simulink model "SAD_project"  (R2023b)
settings: Solver=ode4  StartTime=t0  StopTime=tf  FixedStep=t_step  RelTol=1e-3
model workspace (MAT data in the model file):
  N_order = 1
values from neighbouring files (symbols this model uses):
  A1 = importdata("igrfSg.txt")    [SAD_project_code.m]
  A2 = importdata("igrfSh.txt")    [SAD_project_code.m]
  A_1 = area_face(1)    [SAD_project_code.m]
  A_2 = area_face(2)    [SAD_project_code.m]
  A_3 = area_face(3)    [SAD_project_code.m]
  A_4 = area_face(4)    [SAD_project_code.m]
  A_5 = area_face(5)    [SAD_project_code.m]
  A_6 = area_face(6)    [SAD_project_code.m]
  alpha = [1/6 5/6]    [SAD_project_code.m]
  ARW = ARW*[1 1 1]'    [SAD_project_code.m]
  bias = bias*[1 1 1]'    [SAD_project_code.m]
  DCM_eci_per = rotationMatrix(rad2deg(i),rad2deg(OM), rad2deg(om))    [SAD_project_code.m]
  e = 0.0011241    [SAD_project_code.m]
  FS = 50000e-9    (= 5e-05)    [SAD_project_code.m]
  H0 = [g_10 g_11 h_11]'    [SAD_project_code.m]
  h_r_0 = [0,0,0]'    [SAD_project_code.m]
  horizon_cone_limit = deg2rad(350)    [SAD_project_code.m]
  i = deg2rad(97.55)    [SAD_project_code.m]
  I = 5/12.*diag([Ix Iy Iz])    [SAD_project_code.m]
  I_inv = inv(I)    [SAD_project_code.m]
  I_RW = 1e-2    (= 0.01)    [SAD_project_code.m]
  I_vector_RW = [I_RW I_RW I_RW]'    [SAD_project_code.m]
  inc_tot = sqrt(inc_lin^2 + inc_acc^2)    [SAD_project_code.m]
  InitialTrueAnomalyOfEarth = 0    [SAD_project_code.m]
  j_b = [0.001 0.005 0.001]'    [SAD_project_code.m]
  matrix_RW_config = eye(3)    [SAD_project_code.m]
  matrix_RW_config_inv = inv(matrix_RW_config)    [SAD_project_code.m]
  mu_E = astroConstants(13)    [SAD_project_code.m]
  N_1 = BODY(1,:)    [SAD_project_code.m]
  N_2 = BODY(2,:)    [SAD_project_code.m]
  N_3 = BODY(3,:)    [SAD_project_code.m]
  N_4 = BODY(4,:)    [SAD_project_code.m]
  N_5 = BODY(5,:)    [SAD_project_code.m]
  N_6 = BODY(6,:)    [SAD_project_code.m]
  n_e = sqrt(mu_E/a^3)    [SAD_project_code.m]
  om = deg2rad(206.3209)    [SAD_project_code.m]
  OM = deg2rad(50.7464)    [SAD_project_code.m]
  p = a*(1-e^2)    [SAD_project_code.m]
  q0 = [0.1, -0.7, 0.51, 0.41]    [SAD_project_code.m]
  r_1 = r(1,:)    [SAD_project_code.m]
  r_2 = r(2,:)    [SAD_project_code.m]
  r_3 = r(3,:)    [SAD_project_code.m]
  r_4 = r(4,:)    [SAD_project_code.m]
  r_5 = r(5,:)    [SAD_project_code.m]
  r_6 = r(6,:)    [SAD_project_code.m]
  R_E = astroConstants(23)    [SAD_project_code.m]
  rho_d1 = 0.1    [SAD_project_code.m]
  rho_d2 = 0.1    [SAD_project_code.m]
  rho_d3 = 0.1    [SAD_project_code.m]
  rho_d4 = 0.1    [SAD_project_code.m]
  rho_d5 = 0.1    [SAD_project_code.m]
  rho_d6 = 0.1    [SAD_project_code.m]
  rho_s1 = rho_s(1)    [SAD_project_code.m]
  rho_s2 = rho_s(2)    [SAD_project_code.m]
  rho_s3 = rho_s(3)    [SAD_project_code.m]
  rho_s4 = rho_s(4)    [SAD_project_code.m]
  rho_s5 = rho_s(5)    [SAD_project_code.m]
  rho_s6 = rho_s(6)    [SAD_project_code.m]
  t_step = 0.01    [SAD_project_code.m]
  th0 = deg2rad(0)    [SAD_project_code.m]
  timeoflaunch = date2mjd2000(date0)    [SAD_project_code.m]
  ts_sensor = 5*t_step    (= 0.05)    [SAD_project_code.m]
  w0 = [wx0 wy0 wz0]'    [SAD_project_code.m]
  w0_RW = [0 0 0]    [SAD_project_code.m]
  w_E = deg2rad(15.04)/60/60    [SAD_project_code.m]
  wMax_RW = 2*pi * RPM_max_RW / 60    (= 527.263967027)    [SAD_project_code.m]
libraries: matrix_library x21, simulink x5, simulink_extras x4, dspindex x3, vrlib x2, aerolibutil x1
(part 1 of 3)
settings Model: Creator=samue  LastModifiedBy=rkomiii_masca

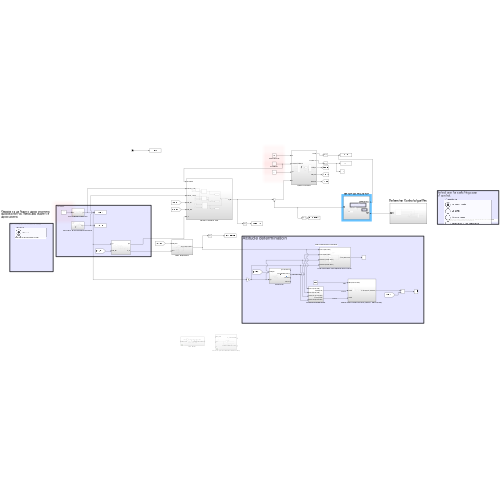
[thumbnail: Simulink's stored preview of the top-level diagram]
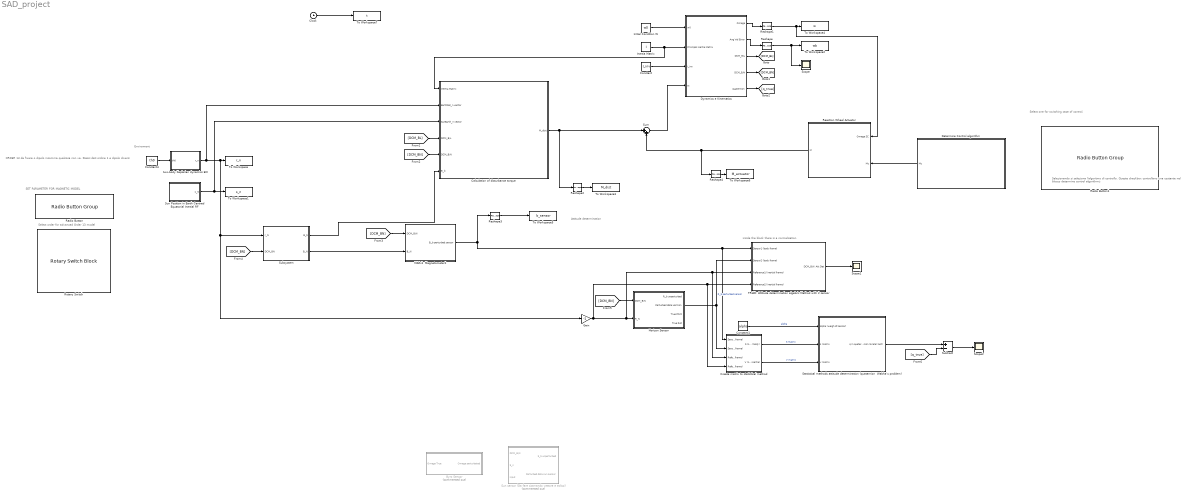
== system SAD_project ==
  note: ORDER 13 da fixare o dipolo insomma qualcosa non va. Stessi dati ordine 1 e dipolo diversi
  note: Select order for advanced Order 13 model
  note: SET PARAMETER FOR MAGNETIC MODEL
  note: Selezionando si seleziona l'algoritmo di controllo. Queste checkbox controllano una costante nel blocco determine control algorithmù
  note: Select one for switching case
      | of control.
  note: Attitude determination
  note: inside the block there is a normalisation
  note: Enviroment
  Calculation of disturbance torque : Subsystem
  Clock : Clock
  Constant : Constant  Value=I_inv
  Constant1 : Constant  Value=alpha
  Constant4 : Constant  Value=th0
  Create matrix to statistical method : Subsystem
  Determine Control algorithm : Subsystem
  Dynamics e Kinematics : Subsystem
  Gain : Gain  Gain=-1
  Gyro Sensor : Subsystem  Commented=on
  Horizon Sensor : Subsystem
  Inertia Matrix : Constant  Value=I  VectorParams1D=off
  Initial Condition W : Constant  Value=w0
  MAG-3  Magnetometer1 : Subsystem
  Radio Button : RadioButtonGroup  LabelPosition=Hide  SelectedLabel=Dipole model  ButtonGroupName=Magnetic field
      settings: Values={{'Dipole model', 'Order 13 model'}, [0 1]}
  Radio Button1 : RadioButtonGroup  LabelPosition=Hide  SelectedLabel=No control mode  ButtonGroupName=Control Mode
      settings: Values={{'No control mode', 'De-tumble', 'Slew maneuver', 'Pointing with 3 axis stabilization'}, [0 1 2 3]}
  Reaction Wheel Actuator : Subsystem
  Reshape{,1..4} (5 alike) : Reshape
  Rotary Switch : RotarySwitchBlock  LabelPosition=Hide
      settings: Values={{'1', '2', '3', '4', '5', '6', '7', '8', '9', '10', '11', '12', '13'}, [1 2 3 4 5 6 7 8 9 10 11 12 13]}
  Scope : Scope
  Scope1 : Scope
  Scope2 : Scope
  "Statistical methods attitude determination (quaternion  Wabha’s problem) " : Subsystem
  Subsystem : Subsystem
  Subtract : Sum  Inputs=+-
  Sum : Sum  Inputs=|++
  Sun Position in Earth Centred Equatorial Inertial RF : Subsystem
  Sun sensor (Da fare sistmando vettore e eclissi) : Subsystem  Commented=on
  TRIAD: Attitude determination algebric Method with 2 sensor : Subsystem
  To Workspace : ToWorkspace  VariableName=r_n  SampleTime=-1
  To Workspace1 : ToWorkspace  VariableName=s_n  SampleTime=-1
  To Workspace2 : ToWorkspace  VariableName=wb  SampleTime=-1
  To Workspace3 : ToWorkspace  VariableName=M_dist  SampleTime=-1
  To Workspace4 : ToWorkspace  VariableName=w  SampleTime=-1
  To Workspace5 : ToWorkspace  VariableName=b_sensor  SampleTime=-1
  To Workspace6 : ToWorkspace  VariableName=M_actuator  SampleTime=-1
  To Workspace7 : ToWorkspace  VariableName=t  SampleTime=-1
  two-body Keplerian dynamics ECI : Subsystem
  wires:
  two-body Keplerian dynamics ECI/1(r_n) -> Calculation of disturbance torque/2(EarthSat_n vector), Gain/1, Subsystem/1(r_N), To Workspace/1
  Inertia Matrix/1 -> Calculation of disturbance torque/1(Inertia Matrix), Dynamics e Kinematics/2(Principal Inertia Matrix)
  Initial Condition W/1 -> Dynamics e Kinematics/1(w0)
  Reshape/1 -> Scope/1, To Workspace2/1
  Dynamics e Kinematics/2(Ang Vel Error) -> Reshape/1
  Dynamics e Kinematics/3(DCM_B/L) -> [DCM_BL]
  Dynamics e Kinematics/1(Omega) -> Reshape1/1
  Constant4/1 -> two-body Keplerian dynamics ECI/1(th0)
  Constant/1 -> Dynamics e Kinematics/3(I_inv)
  Clock/1 -> To Workspace7/1
  Calculation of disturbance torque/1(M_dist) -> Sum/1, Reshape2/1
  [DCM_BN] -> MAG-3  Magnetometer1/1(DCM_B/N)
  [DCM_BL] -> Calculation of disturbance torque/4(DCM_B/L)
  [DCM_BN] -> Calculation of disturbance torque/5(DCM_B/N)
  [DCM_BN] -> Subsystem/2(DCM_BN)
  Reshape1/1 -> Reaction Wheel Actuator/1(Omega SC), To Workspace4/1
  Reshape2/1 -> To Workspace3/1
  Sun Position in Earth Centred Equatorial Inertial RF/1(s_N) -> To Workspace1/1, Calculation of disturbance torque/3(SunEarth_n vector)
  Dynamics e Kinematics/4(DCM_B/N) -> [DCM_BN]
  "Statistical methods attitude determination (quaternion  Wabha’s problem) "/1(q in quaternion (scalar last)) -> Subtract/1
  Create matrix to statistical method/2(V matrix (inertia)) -> "Statistical methods attitude determination (quaternion  Wabha’s problem) "/3(v matrix)  "V matrix"
  Constant1/1 -> "Statistical methods attitude determination (quaternion  Wabha’s problem) "/1(alpha (weigh of sensor))  "alpha"
  Create matrix to statistical method/1(S matrix (body)) -> "Statistical methods attitude determination (quaternion  Wabha’s problem) "/2(s matrix)  "S matrix"
  Horizon Sensor/2(Perturbed data Horizon) -> Create matrix to statistical method/2(Sensor2 (body frame)), TRIAD: Attitude determination algebric Method with 2 sensor/2(Sensor2 (body frame))  "R_b perturbed sensor"
  Gain/1 -> Horizon Sensor/2(R_N), TRIAD: Attitude determination algebric Method with 2 sensor/3(Reference1 (Inertial frame)), Create matrix to statistical method/3(Reference1 (Inertial frame)), TRIAD: Attitude determination algebric Method with 2 sensor/4(Reference2 (Inertial frame)), Create matrix to statistical method/4(Reference2 (Inertial frame))
  Reshape3/1 -> To Workspace5/1
  MAG-3  Magnetometer1/1(B_b perturbed sensor) -> Create matrix to statistical method/1(Sensor1 (body frame)), TRIAD: Attitude determination algebric Method with 2 sensor/1(Sensor1 (body frame)), Reshape3/1
  Subsystem/1(B_b) -> Calculation of disturbance torque/6(B_b)
  Determine Control algorithm/1(Mc) -> Reaction Wheel Actuator/2(Mc)
  Sum/1 -> Dynamics e Kinematics/4(M)
  Subsystem/2(B_N) -> MAG-3  Magnetometer1/2(B_N)
  [DCM_BN] -> Horizon Sensor/1(DCM_B/N)
  TRIAD: Attitude determination algebric Method with 2 sensor/1(DCM_B/N  Att Det) -> Scope1/1
  Dynamics e Kinematics/5(quaternion) -> [q_true]
  [q_true] -> Subtract/2
  Subtract/1 -> Scope2/1
  Reaction Wheel Actuator/1(M) -> Reshape4/1, Sum/2
  Reshape4/1 -> To Workspace6/1

== system SAD_project/Calculation of disturbance torque ==
  Inertia Matrix : Inport
  EarthSat_n vector : Inport  Port=2
  SunEarth_n vector : Inport  Port=3
  DCM_B/L : Inport  Port=4
  DCM_B/N : Inport  Port=5
  B_b : Inport  Port=6
  Extract Diagonal : matrix_library/Extract Diagonal
      settings: LibrarySourceBlock=|
      | simulink/Matrix
      | Operations/Extract Diagonal
  M of gravity gradient1 : Subsystem
  Magnetic Torque : Subsystem
  Reshape : Reshape
  Reshape1 : Reshape
  Solar pressure on 6 faces : Subsystem
  Sum : Sum  Inputs=|+++
  Terminator : Terminator
  To Workspace1 : ToWorkspace  VariableName=M_b  SampleTime=-1
  To Workspace3 : ToWorkspace  VariableName=M_GG  SampleTime=-1
  To Workspace8 : ToWorkspace  VariableName=M_SRP  SampleTime=-1
  j_b : Constant  Value=j_b
  M_dist : Outport
  wires:
  DCM_B/L/1 -> M of gravity gradient1/2(A_B/L)
  j_b/1 -> Magnetic Torque/1(j_b)
  Magnetic Torque/1(M_b) -> Sum/3, Reshape1/1
  B_b/1 -> Magnetic Torque/2(B_b)
  Inertia Matrix/1 -> Extract Diagonal/1
  DCM_B/N/1 -> Solar pressure on 6 faces/1(DCM)
  Sum/1 -> M_dist/1
  Reshape/1 -> To Workspace8/1
  Reshape1/1 -> To Workspace1/1
  M of gravity gradient1/1(GravityGradient_M) -> To Workspace3/1, Sum/1
  Solar pressure on 6 faces/2(Ftot_SP) -> Terminator/1
  Solar pressure on 6 faces/1(Mtot_SP) -> Reshape/1
  Extract Diagonal/1 -> M of gravity gradient1/1(Inertia Vector)
  EarthSat_n vector/1 -> Solar pressure on 6 faces/3("r_N "), M of gravity gradient1/3(r_N)
  SunEarth_n vector/1 -> Solar pressure on 6 faces/2(S_N)

== system SAD_project/Create matrix to statistical method ==
  Sensor1 (body frame) : Inport
  Sensor2 (body frame) : Inport  Port=2
  Reference1 (Inertial frame) : Inport  Port=3
  Reference2 (Inertial frame) : Inport  Port=4
  Matrix Concatenate1 : Concatenate  Mode=Multidimensional array  ConcatenateDimension=2
  Matrix Concatenate2 : Concatenate  Mode=Multidimensional array  ConcatenateDimension=2
  Normalize Vector1 : Subsystem
  Normalize Vector2 : Subsystem
  Normalize Vector3 : Subsystem
  Normalize Vector4 : Subsystem
  S matrix (body) : Outport
  V matrix (inertia) : Outport  Port=2
  wires:
  Matrix Concatenate1/1 -> V matrix (inertia)/1
  Normalize Vector1/1(Versor) -> Matrix Concatenate2/1
  Normalize Vector2/1(Versor) -> Matrix Concatenate2/2
  Normalize Vector4/1(Versor) -> Matrix Concatenate1/2
  Normalize Vector3/1(Versor) -> Matrix Concatenate1/1
  Matrix Concatenate2/1 -> S matrix (body)/1
  Reference1 (Inertial frame)/1 -> Normalize Vector3/1(Vector)
  Reference2 (Inertial frame)/1 -> Normalize Vector4/1(Vector)
  Sensor1 (body frame)/1 -> Normalize Vector1/1(Vector)
  Sensor2 (body frame)/1 -> Normalize Vector2/1(Vector)

== system SAD_project/Determine Control algorithm ==
  note: Modificare i case Switch case action tranquillamente aggiungendo tutti gli input desiderati
  Constant : Constant  Value=[1;1;1]
  Constant1 : Constant  Value=[2;2;2]
  Constant2 : Constant  Value=0
  Constant3 : Constant  Value=[3;3;3]
  Merge : Merge  Inputs=4
  Switch Case : SwitchCase  CaseConditions={1,2,3}
  Switch Case Action 3 axis stabilization Algorithm : Subsystem  TreatAsAtomicUnit=on
  Switch Case Action Detumle Algorithm : Subsystem  TreatAsAtomicUnit=on
  Switch Case Action Mc = 0 : Subsystem  TreatAsAtomicUnit=on
  Switch Case Action Slew Maneuver Algorithm : Subsystem  TreatAsAtomicUnit=on
  Mc : Outport
  wires:
  Switch Case/2 -> Switch Case Action Slew Maneuver Algorithm/Action  "slew maneuver"
  Switch Case/1 -> Switch Case Action Detumle Algorithm/Action  "Detumble case"
  Switch Case Action Slew Maneuver Algorithm/1(Out1) -> Merge/2
  Switch Case/3 -> Switch Case Action 3 axis stabilization Algorithm/Action  "pointing with 3 axis stabilization"
  Switch Case Action Mc = 0/1(Output) -> Merge/4
  Constant2/1 -> Switch Case/1
  Switch Case Action Detumle Algorithm/1(Output) -> Merge/1
  Switch Case Action 3 axis stabilization Algorithm/1(Out1) -> Merge/3
  Switch Case/4 -> Switch Case Action Mc = 0/Action  "Default: Contol moment == 0"
  Merge/1 -> Mc/1  "Control Moment"
  Constant/1 -> Switch Case Action Detumle Algorithm/1(Input)
  Constant1/1 -> Switch Case Action Slew Maneuver Algorithm/1(In1)
  Constant3/1 -> Switch Case Action 3 axis stabilization Algorithm/1(In1)

== system SAD_project/Dynamics e Kinematics ==
  w0 : Inport
  Principal Inertia Matrix : Inport  Port=2
  I_inv : Inport  Port=3
  M : Inport  Port=4
  Attitude error GG : Subsystem
  Constant6 : Constant  Value=q0
  DCM composition from quaternions 1 : Subsystem  AncestorBlock=LibrarySAD5/DCM composition from quaternions
  Kinematics quaternion2 : Subsystem
  Single spin dynamics : Subsystem  AncestorBlock=My_library/Single spin dynamics
  Terminator1 : Terminator
  Omega : Outport
  Ang Vel Error : Outport  Port=2
  DCM_B/L : Outport  Port=3
  DCM_B/N : Outport  Port=4
  quaternion : Outport  Port=5
  wires:
  DCM composition from quaternions 1/1(DCM) -> DCM_B/N/1, Attitude error GG/2(DCM_B/N)
  Constant6/1 -> Kinematics quaternion2/2(q0)
  Single spin dynamics/1(Omega) -> Omega/1, Attitude error GG/1(w), Kinematics quaternion2/1(omega)
  Kinematics quaternion2/2(q^(-1)) -> Terminator1/1
  M/1 -> Single spin dynamics/4(M)
  w0/1 -> Single spin dynamics/3(Omega_0)
  Principal Inertia Matrix/1 -> Single spin dynamics/2(Inertia matrix)
  Kinematics quaternion2/1(q) -> quaternion/1, DCM composition from quaternions 1/1(q(4x1))
  Attitude error GG/2(DCM_B/L) -> DCM_B/L/1
  Attitude error GG/1(Ang Vel Error) -> Ang Vel Error/1
  I_inv/1 -> Single spin dynamics/1(Inertia matrix inverse)

== system SAD_project/Gyro Sensor ==
  Omega True : Inport
  Band-Limited White Noise : simulink/Sources/Band-Limited White Noise  Cov=[0.00001]  Ts=0.1  seed=[23341]
  Constant : Constant  Value=ARW  VectorParams1D=off
  Constant1 : Constant  Value=bias  VectorParams1D=off
  Sum : Sum  Inputs=|++
  Sum1 : Sum  Inputs=|++
  Sum2 : Sum  Inputs=|++
  Zero-Order Hold : ZeroOrderHold  SampleTime=-1
  Omega perturbated : Outport
  wires:
  Zero-Order Hold/1 -> Sum/1
  Sum2/1 -> Omega perturbated/1
  Sum1/1 -> Sum2/1
  Sum/1 -> Sum1/1
  Omega True/1 -> Zero-Order Hold/1
  Constant1/1 -> Sum2/2
  Band-Limited White Noise/1 -> Sum/2
  Constant/1 -> Sum1/2

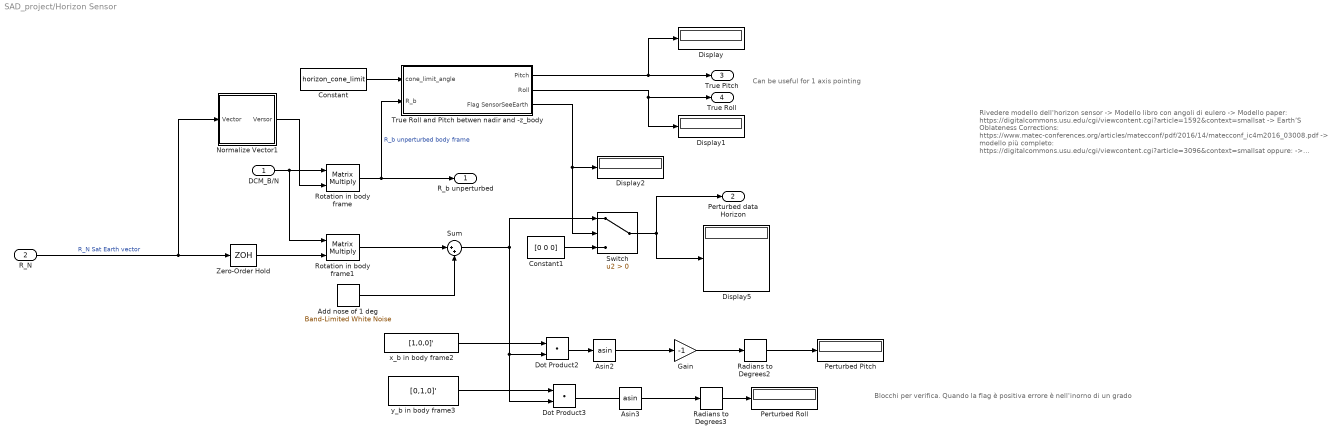
== system SAD_project/Horizon Sensor ==
  note: Can be useful for 1 axis pointing
  note: Rivedere modello dell'horizon sensor
      | -> Modello libro con angoli di eulero
      | -> Modello paper: https://digitalcommons.usu.edu/cgi/viewcontent.cgi?article=1592&context=smallsat
      | -> Earth’S Oblateness Corrections: https://www.matec-conferences.org/articles/matecconf/pdf/2016/14/matecconf_ic4m2016_03008.pdf
      | -> modello più completo: https://digitalcommons.usu.edu/cgi/viewcontent.cgi?article=3096&context=smallsat
      | oppure:
      | -> Sistemare errore in modo che non sia lineare
      | -> Controllare angoli e conversioni
  note: Blocchi per verifica. Quando la flag è positiva errore è nell'inorno di un grado
  DCM_B/N : Inport
  R_N : Inport  Port=2
  Add nose of 1 deg : simulink/Sources/Band-Limited White Noise  Cov=[0.000001 0.000001 0]  Ts=ts_sensor  seed=[23341]
  Asin2 : Trigonometry  Operator=asin
  Asin3 : Trigonometry  Operator=asin
  Constant : Constant  Value=horizon_cone_limit
  Constant1 : Constant  Value=[0 0 0]
  Display{,1..2,5} (4 alike) : Display
  Dot Product2 : DotProduct  OutDataTypeStr=Inherit: Inherit via internal rule
  Dot Product3 : DotProduct  OutDataTypeStr=Inherit: Inherit via internal rule
  Gain : Gain  Gain=-1
  Normalize Vector1 : Subsystem
  Perturbed Pitch : Display
  Perturbed Roll : Display
  Radians to Degrees2 : simulink_extras/Transformations/Radians to Degrees
  Radians to Degrees3 : simulink_extras/Transformations/Radians to Degrees
  Rotation in body frame : Product  Multiplication=Matrix(*)
  Rotation in body frame1 : Product  Multiplication=Matrix(*)
  Sum : Sum  Inputs=|++
  Switch : Switch  Criteria=u2 > Threshold  SaturateOnIntegerOverflow=off  InputSameDT=off
  True Roll and Pitch betwen nadir and -z_body : Subsystem
  Zero-Order Hold : ZeroOrderHold  SampleTime=ts_sensor
  x_b in body frame2 : Constant  Value=[1,0,0]'
  y_b in body frame3 : Constant  Value=[0,1,0]'
  R_b unperturbed : Outport
  Perturbed data Horizon : Outport  Port=2
  True Pitch : Outport  Port=3
  True Roll : Outport  Port=4
  wires:
  y_b in body frame3/1 -> Dot Product3/1
  Zero-Order Hold/1 -> Rotation in body frame1/2
  True Roll and Pitch betwen nadir and -z_body/3(Flag SensorSeeEarth) -> Switch/2, Display2/1
  Normalize Vector1/1(Versor) -> Rotation in body frame/2
  Rotation in body frame1/1 -> Sum/1
  Asin2/1 -> Gain/1
  DCM_B/N/1 -> Rotation in body frame/1, Rotation in body frame1/1
  Switch/1 -> Perturbed data Horizon/1, Display5/1
  True Roll and Pitch betwen nadir and -z_body/1(Pitch) -> Display/1, True Pitch/1
  Constant/1 -> True Roll and Pitch betwen nadir and -z_body/1(cone_limit_angle)
  Dot Product2/1 -> Asin2/1
  Rotation in body frame/1 -> R_b unperturbed/1, True Roll and Pitch betwen nadir and -z_body/2(R_b)  "R_b unperturbed body frame"
  Add nose of 1 deg/1 -> Sum/2
  True Roll and Pitch betwen nadir and -z_body/2(Roll) -> Display1/1, True Roll/1
  x_b in body frame2/1 -> Dot Product2/1
  Radians to Degrees2/1 -> Perturbed Pitch/1
  Sum/1 -> Switch/1, Dot Product2/2, Dot Product3/2
  Dot Product3/1 -> Asin3/1
  Asin3/1 -> Radians to Degrees3/1
  Gain/1 -> Radians to Degrees2/1
  Radians to Degrees3/1 -> Perturbed Roll/1
  Constant1/1 -> Switch/3
  R_N/1 -> Zero-Order Hold/1, Normalize Vector1/1(Vector)  "R_N Sat Earth vector"

== system SAD_project/MAG-3  Magnetometer1 ==
  note: CODE TO ADD TO MAKE SENSOR WORK
      | % Time definition
      | t0 = 0;
      | tf = T; %Period of orbit
      | t_step = 0.01; %fixed step of simulation
      | ts_sensor = t_step; % Sample of sensor (can change but must to be a multiple of t_step)
      |
      | % MAG-3 sensor data and error
      | FS = 500e-9; %Full scale value
      | inc_lin = 0.15/100; % Accuracy error
      | inc_acc = 0.75/100; % Linear error
      | inc_tot = sqrt(inc_lin^2 + inc_acc^2); %Total error
  DCM_B/N : Inport
  B_N : Inport  Port=2
  Error gain of sensor MAG-3 : Gain  Gain=inc_tot*FS
  Rotation in body frame : Product  Multiplication=Matrix(*)
  Saturation to FS : Saturate  UpperLimit=FS  LowerLimit=-FS
  Sum : Sum  Inputs=|++
  Vector Concatenate : Concatenate  NumInputs=3
  White Noise : RandomNumber  DisableCoverage=on  Seed=1  SampleTime=ts_sensor
  White Noise1 : RandomNumber  DisableCoverage=on  Seed=2  SampleTime=ts_sensor
  White Noise2 : RandomNumber  DisableCoverage=on  Seed=3  SampleTime=ts_sensor
  Zero-Order Hold : ZeroOrderHold  SampleTime=ts_sensor
  B_b perturbed sensor : Outport
  wires:
  Vector Concatenate/1 -> Error gain of sensor MAG-3/1
  White Noise/1 -> Vector Concatenate/1
  Error gain of sensor MAG-3/1 -> Sum/2
  White Noise2/1 -> Vector Concatenate/3
  White Noise1/1 -> Vector Concatenate/2
  DCM_B/N/1 -> Rotation in body frame/1
  B_N/1 -> Zero-Order Hold/1
  Zero-Order Hold/1 -> Rotation in body frame/2
  Saturation to FS/1 -> B_b perturbed sensor/1
  Rotation in body frame/1 -> Sum/1
  Sum/1 -> Saturation to FS/1

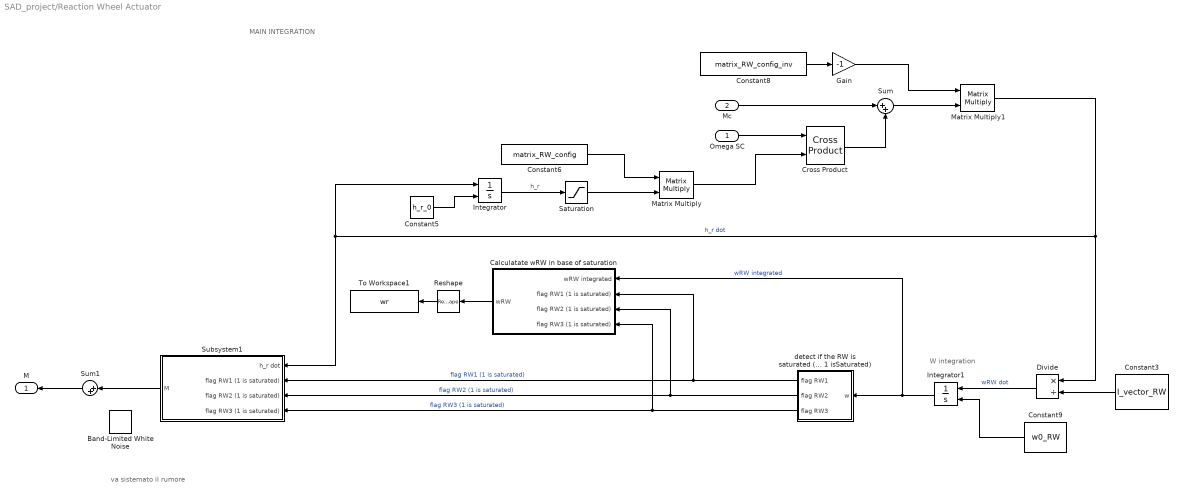
== system SAD_project/Reaction Wheel Actuator ==
  note: W integration
  note: va sistemato il rumore
  note: MAIN INTEGRATION
  Omega SC : Inport
  Mc : Inport  Port=2
  Band-Limited White Noise : simulink/Sources/Band-Limited White Noise  Cov=[0.00001, 0.00001, 0.00001]'  Ts=t_step  seed=[23341]
  Calculatate wRW in base of saturation : Subsystem
  Constant3 : Constant  Value=I_vector_RW
  Constant5 : Constant  Value=h_r_0  VectorParams1D=off
  Constant6 : Constant  Value=matrix_RW_config  VectorParams1D=off
  Constant8 : Constant  Value=matrix_RW_config_inv  VectorParams1D=off
  Constant9 : Constant  Value=w0_RW
  Cross Product : matrix_library/Cross Product
  Divide : Product  Inputs=*/
  Gain : Gain  Gain=-1
  Integrator : Integrator  InitialConditionSource=external
  Integrator1 : Integrator  InitialConditionSource=external
  Matrix Multiply : Product  Multiplication=Matrix(*)
  Matrix Multiply1 : Product  Multiplication=Matrix(*)
  Reshape : Reshape
  Saturation : Saturate  UpperLimit=wMax_RW*I_RW  LowerLimit=-wMax_RW*I_RW
  Subsystem1 : Subsystem
  Sum : Sum  Inputs=|++
  Sum1 : Sum  Inputs=|++
  To Workspace1 : ToWorkspace  VariableName=wr  SampleTime=-1
  detect if the RW is saturated (output == 1 isSaturated) : Subsystem
  M : Outport
  wires:
  Matrix Multiply1/1 -> Integrator/1, Subsystem1/1(h_r dot), Divide/1  "h_r dot"
  Constant6/1 -> Matrix Multiply/1
  Cross Product/1 -> Sum/2
  Constant8/1 -> Gain/1
  Sum/1 -> Matrix Multiply1/2
  detect if the RW is saturated (output == 1 isSaturated)/2(flag RW2) -> Calculatate wRW in base of saturation/3(flag RW2 (1 is saturated)), Subsystem1/3(flag RW2 (1 is saturated))  "flag RW2 (1 is saturated)"
  Calculatate wRW in base of saturation/1(wRW) -> Reshape/1
  Matrix Multiply/1 -> Cross Product/2
  Constant5/1 -> Integrator/2
  Constant3/1 -> Divide/2
  Gain/1 -> Matrix Multiply1/1
  Mc/1 -> Sum/1
  Saturation/1 -> Matrix Multiply/2
  Integrator1/1 -> Calculatate wRW in base of saturation/1(wRW integrated), detect if the RW is saturated (output == 1 isSaturated)/1(w)  "wRW integrated"
  Constant9/1 -> Integrator1/2
  Divide/1 -> Integrator1/1  "wRW dot"
  Integrator/1 -> Saturation/1  "h_r"
  detect if the RW is saturated (output == 1 isSaturated)/3(flag RW3) -> Calculatate wRW in base of saturation/4(flag RW3 (1 is saturated)), Subsystem1/4(flag RW3 (1 is saturated))  "flag RW3 (1 is saturated)"
  detect if the RW is saturated (output == 1 isSaturated)/1(flag RW1) -> Calculatate wRW in base of saturation/2(flag RW1 (1 is saturated)), Subsystem1/2(flag RW1 (1 is saturated))  "flag RW1 (1 is saturated)"
  Reshape/1 -> To Workspace1/1
  Omega SC/1 -> Cross Product/1
  Subsystem1/1(M) -> Sum1/1
  Sum1/1 -> M/1

== system SAD_project/Statistical methods attitude determination (quaternion  Wabha’s problem)  ==
  note: In questo blocco ci sono altri metodi per il calcolo di q
  note: BLOCCO DA SISTEMARE SCEGLIENDO UNA SOLUZIONE
  note: Resolve linear system:
      | (𝑆 − σI)𝑞 + zq_4 = 𝜆_(MAX)*𝑞
      | 𝑧'𝑞 + σ*q_4 = 𝜆_(MAX)*𝑞_4
      |
      | Calculate eigenvalue (in the theory we assumed that lambda_max = 1)
  note: 𝐾 = [ (𝑆 − σI), 𝑧
      | 𝑧 ' 𝜎 ]
  note: 𝑧 = [𝑏23 − 𝑏32 , b31 − 𝑏13 , b12 − 𝑏21] '
  alpha (weigh of sensor) : Inport
  s matrix : Inport  Port=2
  v matrix : Inport  Port=3
  Adjoint of 3x3 Matrix : aerolibutil/Adjoint of 3x3 Matrix
  Blocco da convertire in formato simulink. Ho trovato 3 soluzioni differenti al proble : MATLAB Function  TreatAsAtomicUnit=on
  For Iterator Subsystem to calculate B matrix : Subsystem  TreatAsAtomicUnit=on
  Gain : Gain  Gain=eye(3)
  Matrix Concatenate : Concatenate  Mode=Multidimensional array  ConcatenateDimension=2
  Matrix Concatenate1 : Concatenate  Mode=Multidimensional array
  Matrix trace : Subsystem
  Subtract : Sum  Inputs=+-
  Sum : Sum  Inputs=|++
  Transpose : Math  Operator=transpose
  Transpose2 : Math  Operator=transpose
  Vector Concatenate1 : Concatenate
  Vector z : Subsystem
  q in quaternion (scalar last) : Outport
  wires:
  Transpose/1 -> Sum/2
  For Iterator Subsystem to calculate B matrix/1(B matrix) -> Vector z/1(B), Matrix trace/1(Matrix), Transpose/1, Sum/1  "B matrix"
  Sum/1 -> Adjoint of 3x3 Matrix/1, Blocco da convertire in formato simulink. Ho trovato 3 soluzioni differenti al proble/2(S), Subtract/1  "matrix S"
  Gain/1 -> Subtract/2
  Matrix trace/1(trace) -> Vector Concatenate1/2, Gain/1  "sigma = tr(B)"
  Matrix Concatenate/1 -> Matrix Concatenate1/1
  Vector Concatenate1/1 -> Transpose2/1
  Vector z/1(z) -> Vector Concatenate1/1, Matrix Concatenate/2
  Transpose2/1 -> Matrix Concatenate1/2
  Subtract/1 -> Matrix Concatenate/1  "S - sigma*eye(3)"
  alpha (weigh of sensor)/1 -> For Iterator Subsystem to calculate B matrix/1(alpha)
  v matrix/1 -> For Iterator Subsystem to calculate B matrix/3(v matrix)
  s matrix/1 -> For Iterator Subsystem to calculate B matrix/2(s matrix)
  Blocco da convertire in formato simulink. Ho trovato 3 soluzioni differenti al proble/1(q) -> q in quaternion (scalar last)/1  "q in quaternion (scalar last)"
  Adjoint of 3x3 Matrix/1 -> Blocco da convertire in formato simulink. Ho trovato 3 soluzioni differenti al proble/3(Sadj)
  Matrix Concatenate1/1 -> Blocco da convertire in formato simulink. Ho trovato 3 soluzioni differenti al proble/1(K)  "K matrix"

== system SAD_project/Subsystem ==
  r_N : Inport
  DCM_BN : Inport  Port=2
  Control by check box : Constant  Value=0
  Matrix Multiply : Product  Multiplication=Matrix(*)
  Merge : Merge
  Reshape4 : Reshape
  Switch Case Action Adavanced Magnetic model : Subsystem  TreatAsAtomicUnit=on
  Switch Case Action Dipole model : Subsystem  TreatAsAtomicUnit=on
  Switch Case2 : SwitchCase
  To Workspace6 : ToWorkspace  VariableName=bn  SampleTime=-1
  B_b : Outport
  B_N : Outport  Port=2
  wires:
  Switch Case Action Dipole model/1(b_N) -> Merge/2
  Switch Case2/1 -> Switch Case Action Adavanced Magnetic model/Action
  Switch Case2/2 -> Switch Case Action Dipole model/Action
  Matrix Multiply/1 -> B_b/1
  DCM_BN/1 -> Matrix Multiply/1
  Control by check box/1 -> Switch Case2/1
  r_N/1 -> Switch Case Action Dipole model/1(r_N), Switch Case Action Adavanced Magnetic model/1(r_N)
  Switch Case Action Adavanced Magnetic model/1(B_n) -> Merge/1
  Reshape4/1 -> To Workspace6/1
  Merge/1 -> Reshape4/1, Matrix Multiply/2, B_N/1

== system SAD_project/Sun Position in Earth Centred Equatorial Inertial RF ==
  note: pointing Sun from Earth
      |
      | x=vernal line
      | y=perpendicular
      | z=cnp
  Clock : Clock
  Gain : Gain  Gain=cos(23.45/360*2*pi)
  Gain1 : Gain  Gain=sin(23.45/360*2*pi)
  InitialTrueAnomalyOfEarth : Constant  Value=InitialTrueAnomalyOfEarth
  MatrixMultiply : Product
  Mux : Mux  Inputs=3
  Product : Product
  Sum : Sum  Inputs=|++
  Trigonometric Function : Trigonometry  Operator=cos
  Trigonometric Function1 : Trigonometry
  mean ang vel : Constant  Value=2*pi/31536000
  mean distance : Constant  Value=149597870
  s_N : Outport
  wires:
  Trigonometric Function/1 -> Mux/1
  Gain1/1 -> Mux/3
  Mux/1 -> MatrixMultiply/2
  MatrixMultiply/1 -> s_N/1  "s_N"
  mean distance/1 -> MatrixMultiply/1
  Gain/1 -> Mux/2
  Trigonometric Function1/1 -> Gain1/1, Gain/1
  mean ang vel/1 -> Product/2
  Clock/1 -> Product/1
  InitialTrueAnomalyOfEarth/1 -> Sum/2
  Product/1 -> Sum/1
  Sum/1 -> Trigonometric Function1/1, Trigonometric Function/1

== system SAD_project/Sun sensor (Da fare sistmando vettore e eclissi) ==
  note: SUN SENSOR DA RIFINIRE, ma Utilizzabile
      | -> Modellare non rilevamento sole (esempio eclissi)
      | -> Modellare albedo terra/luna per riflessi
      | -> Sistemare distrubi basandosi su sensore reale
  DCM_B/N : Inport
  S_n : Inport  Port=2
  Input : Inport  Port=3
  Band-Limited White Noise : simulink/Sources/Band-Limited White Noise  Cov=5e9*[1 1 1]  Ts=ts_sensor  seed=[23341]
  Normalize Vector1 : Subsystem
  Rotation in body frame : Product  Multiplication=Matrix(*)
  Rotation in body frame1 : Product  Multiplication=Matrix(*)
  Sum : Sum  Inputs=|++
  Zero-Order Hold : ZeroOrderHold  SampleTime=ts_sensor
  S_b unperturbed : Outport
  Perturbed data sun sensor : Outport  Port=2
  wires:
  Band-Limited White Noise/1 -> Sum/2
  DCM_B/N/1 -> Rotation in body frame/1, Rotation in body frame1/1
  S_n/1 -> Zero-Order Hold/1, Normalize Vector1/1(Vector)
  Normalize Vector1/1(Versor) -> Rotation in body frame/2
  Zero-Order Hold/1 -> Rotation in body frame1/2
  Rotation in body frame1/1 -> Sum/1
  Rotation in body frame/1 -> S_b unperturbed/1
  Sum/1 -> Perturbed data sun sensor/1

== system SAD_project/TRIAD: Attitude determination algebric Method with 2 sensor ==
  note: 𝑉^(-1) = 𝑉';
      | 𝐴 = 𝑆𝑉^(-1) = 𝑆𝑉'
  note: 𝑣1 = 𝑎;
      | 𝑣2 = (𝑎 ∧ 𝑏)/|𝑎 ∧ 𝑏|;
      | 𝑣3 = 𝑎 ∧ 𝑣2
  note: S1 = 𝑝;
      | 𝑠2 = (𝑝 ∧ 𝑞)/(|𝑝 ∧ 𝑞|);
      | 𝑠3 = 𝑝 ∧ 𝑠2
  Sensor1 (body frame) : Inport
  Sensor2 (body frame) : Inport  Port=2
  Reference1 (Inertial frame) : Inport  Port=3
  Reference2 (Inertial frame) : Inport  Port=4
  Matrix Multiply : Product  Multiplication=Matrix(*)
  Normalize Vector1 : Subsystem
  Normalize Vector2 : Subsystem
  Normalize Vector3 : Subsystem
  Normalize Vector4 : Subsystem
  Subsystem : Subsystem
  Subsystem1 : Subsystem
  Transpose : Math  Operator=transpose
  DCM_B/N  Att Det : Outport
  wires:
  Sensor1 (body frame)/1 -> Normalize Vector2/1(Vector)  "q"
  Sensor2 (body frame)/1 -> Normalize Vector3/1(Vector)  "p"
  Subsystem/1("Matrix S Measurements ") -> Matrix Multiply/1  "Matrix S Measurements (body frame)"
  Normalize Vector2/1(Versor) -> Subsystem/1(versor p (body frame))
  Normalize Vector3/1(Versor) -> Subsystem/2(versor q (body frame))
  Normalize Vector1/1(Versor) -> Subsystem1/1(versor a (body frame))
  Reference2 (Inertial frame)/1 -> Normalize Vector4/1(Vector)  "b"
  Reference1 (Inertial frame)/1 -> Normalize Vector1/1(Vector)  "a"
  Subsystem1/1("Matrix V certain model ") -> Transpose/1  "Matrix V (inertial frame)"
  Normalize Vector4/1(Versor) -> Subsystem1/2(versor b (body frame))
  Matrix Multiply/1 -> DCM_B/N  Att Det/1  "DCM_B/N from attirude determination"
  Transpose/1 -> Matrix Multiply/2

== system SAD_project/two-body Keplerian dynamics ECI ==
  th0 : Inport
  Constant : Constant  Value=DCM_eci_per
  Integretion of true anomaly : Subsystem
  Matrix Multiply : Product  Multiplication=Matrix(*)
  Transpose : Math  Operator=transpose
  r_perifocal : Subsystem
  r_n : Outport
  wires:
  th0/1 -> Integretion of true anomaly/1(th0)
  Integretion of true anomaly/1(th) -> r_perifocal/1(th)
  Constant/1 -> Transpose/1
  Transpose/1 -> Matrix Multiply/1
  r_perifocal/1(r_per) -> Matrix Multiply/2
  Matrix Multiply/1 -> r_n/1

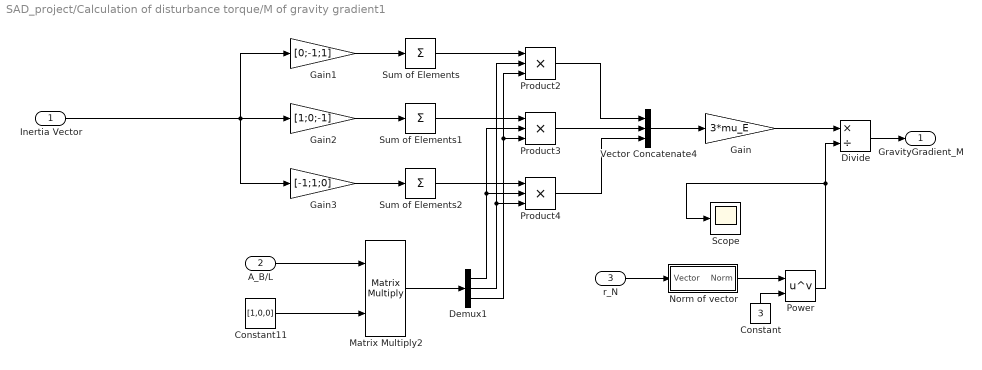
== system SAD_project/Calculation of disturbance torque/M of gravity gradient1 ==
  Inertia Vector : Inport
  A_B/L : Inport  Port=2
  r_N : Inport  Port=3
  Constant : Constant  Value=3
  Constant11 : Constant  Value=[1,0,0]
  Demux1 : Demux  Outputs=3
  Divide : Product  Inputs=*/
  Gain : Gain  Gain=3*mu_E
  Gain1 : Gain  Gain=[0;-1;1]
  Gain2 : Gain  Gain=[1;0;-1]
  Gain3 : Gain  Gain=[-1;1;0]
  Matrix Multiply2 : Product  Multiplication=Matrix(*)
  Norm of vector : Subsystem  AncestorBlock=LibrarySAD5/Normalize Vector1
  Power : Math  Operator=pow
  Product2 : Product  Inputs=3
  Product3 : Product  Inputs=3
  Product4 : Product  Inputs=3
  Scope : Scope
  Sum of Elements : Sum  Inputs=+
  Sum of Elements1 : Sum  Inputs=+
  Sum of Elements2 : Sum  Inputs=+
  Vector Concatenate4 : Concatenate  NumInputs=3
  GravityGradient_M : Outport
  wires:
  Demux1/3 -> Product2/3, Product3/3
  Product2/1 -> Vector Concatenate4/1
  Matrix Multiply2/1 -> Demux1/1
  Product4/1 -> Vector Concatenate4/3
  Product3/1 -> Vector Concatenate4/2
  Demux1/1 -> Product4/2, Product3/2
  Constant11/1 -> Matrix Multiply2/2
  Demux1/2 -> Product4/3, Product2/2
  A_B/L/1 -> Matrix Multiply2/1
  Vector Concatenate4/1 -> Gain/1
  Gain1/1 -> Sum of Elements/1
  Gain2/1 -> Sum of Elements1/1
  Gain3/1 -> Sum of Elements2/1
  Sum of Elements/1 -> Product2/1
  Sum of Elements1/1 -> Product3/1
  Sum of Elements2/1 -> Product4/1
  Inertia Vector/1 -> Gain1/1, Gain2/1, Gain3/1
  Gain/1 -> Divide/1
  Power/1 -> Scope/1, Divide/2
  Constant/1 -> Power/2
  r_N/1 -> Norm of vector/1(Vector)
  Divide/1 -> GravityGradient_M/1
  Norm of vector/1(Norm) -> Power/1

== system SAD_project/Calculation of disturbance torque/Magnetic Torque ==
  j_b : Inport
  B_b : Inport  Port=2
  Cross Product : matrix_library/Cross Product
  M_b : Outport
  wires:
  Cross Product/1 -> M_b/1
  j_b/1 -> Cross Product/1
  B_b/1 -> Cross Product/2

== system SAD_project/Calculation of disturbance torque/Solar pressure on 6 faces ==
  DCM : Inport
  S_N : Inport  Port=2
  "r_N " : Inport  Port=3
  Acos : Trigonometry  Operator=acos
  Dot Product : DotProduct  OutDataTypeStr=Inherit: Inherit via internal rule
  MatrixMultiply : Product  Multiplication=Matrix(*)
  MatrixMultiply1 : Product  Multiplication=Matrix(*)
  Norm of vector : Subsystem  AncestorBlock=LibrarySAD5/Normalize Vector1
  Normalize Vector : vrlib/Utilities/Normalize Vector  maxzero=0
  Normalize Vector1 : vrlib/Utilities/Normalize Vector  maxzero=0
  Solar pressure on 6 faces1 : Subsystem
  Sum1 : Sum  Inputs=|+-
  Mtot_SP : Outport
  Ftot_SP : Outport  Port=2
  wires:
  DCM/1 -> MatrixMultiply1/1, MatrixMultiply/1
  S_N/1 -> Norm of vector/1(Vector), Sum1/1, MatrixMultiply/2, Normalize Vector1/1
  "r_N "/1 -> Sum1/2, MatrixMultiply1/2
  MatrixMultiply1/1 -> Solar pressure on 6 faces1/2(r_B)
  Norm of vector/1(Norm) -> Solar pressure on 6 faces1/5(s_N norm)
  MatrixMultiply/1 -> Solar pressure on 6 faces1/1(s_B)
  Sum1/1 -> Solar pressure on 6 faces1/4(S_N - r_N), Normalize Vector/1
  Normalize Vector/1 -> Dot Product/1
  Normalize Vector1/1 -> Dot Product/2
  Solar pressure on 6 faces1/1(Ftot_SP) -> Ftot_SP/1
  Dot Product/1 -> Acos/1
  Acos/1 -> Solar pressure on 6 faces1/3(S/E_S/sc_angle)
  Solar pressure on 6 faces1/2(Mtot_SP) -> Mtot_SP/1

== system SAD_project/Create matrix to statistical method/Normalize Vector1 ==
  Vector : Inport
  Divide : Product  Inputs=*/
  Normalize Vector : Subsystem  AncestorBlock=LibrarySAD5/Normalize Vector1
  Versor : Outport
  wires:
  Vector/1 -> Normalize Vector/1(Vector), Divide/1
  Divide/1 -> Versor/1
  Normalize Vector/1(Norm) -> Divide/2

== system SAD_project/Create matrix to statistical method/Normalize Vector2 ==
  Vector : Inport
  Divide : Product  Inputs=*/
  Normalize Vector : Subsystem  AncestorBlock=LibrarySAD5/Normalize Vector1
  Versor : Outport
  wires:
  Vector/1 -> Normalize Vector/1(Vector), Divide/1
  Divide/1 -> Versor/1
  Normalize Vector/1(Norm) -> Divide/2

== system SAD_project/Create matrix to statistical method/Normalize Vector3 ==
  Vector : Inport
  Divide : Product  Inputs=*/
  Normalize Vector : Subsystem  AncestorBlock=LibrarySAD5/Normalize Vector1
  Versor : Outport
  wires:
  Vector/1 -> Normalize Vector/1(Vector), Divide/1
  Divide/1 -> Versor/1
  Normalize Vector/1(Norm) -> Divide/2

== system SAD_project/Create matrix to statistical method/Normalize Vector4 ==
  Vector : Inport
  Divide : Product  Inputs=*/
  Normalize Vector : Subsystem  AncestorBlock=LibrarySAD5/Normalize Vector1
  Versor : Outport
  wires:
  Vector/1 -> Normalize Vector/1(Vector), Divide/1
  Divide/1 -> Versor/1
  Normalize Vector/1(Norm) -> Divide/2

== system SAD_project/Determine Control algorithm/Switch Case Action 3 axis stabilization Algorithm ==
  In1 : Inport
  Action Port : ActionPort  ActionPortLabel=case [ 3 ]:
  Out1 : Outport
  wires:
  In1/1 -> Out1/1

== system SAD_project/Determine Control algorithm/Switch Case Action Detumle Algorithm ==
  Input : Inport
  Action Port : ActionPort  PropagateVarSize=During execution  ActionPortLabel=case [ 1 ]:
  Output : Outport
  wires:
  Input/1 -> Output/1

== system SAD_project/Determine Control algorithm/Switch Case Action Mc = 0 ==
  Action Port : ActionPort  PropagateVarSize=During execution  ActionPortLabel=default:
  Constant : Constant  Value=[0 0 0]'
  Output : Outport
  wires:
  Constant/1 -> Output/1

== system SAD_project/Determine Control algorithm/Switch Case Action Slew Maneuver Algorithm ==
  In1 : Inport
  Action Port : ActionPort  ActionPortLabel=case [ 2 ]:
  Out1 : Outport
  wires:
  In1/1 -> Out1/1

== system SAD_project/Dynamics e Kinematics/Attitude error GG ==
  w : Inport
  DCM_B/N : Inport  Port=2
  Clock : Clock
  Constant : Constant  Value=n_e
  Constant5 : Constant  Value=0
  Matrix Multiply1 : Product  Multiplication=Matrix(*)
  Product : Product
  Subtract : Sum  Inputs=+-
  Vector Concatenate3 : Concatenate  NumInputs=3
  calculating A_B/L : Subsystem
  Ang Vel Error : Outport
  DCM_B/L : Outport  Port=2
  wires:
  Constant5/1 -> Vector Concatenate3/2, Vector Concatenate3/1
  Vector Concatenate3/1 -> Matrix Multiply1/2  "w_L/N"
  calculating A_B/L/1(A_B/L) -> Matrix Multiply1/1, DCM_B/L/1
  Matrix Multiply1/1 -> Subtract/2  "A_B/L * w_L/N"
  w/1 -> Subtract/1
  Subtract/1 -> Ang Vel Error/1
  Product/1 -> calculating A_B/L/1(Theta)  "Theta"
  Clock/1 -> Product/2
  Constant/1 -> Product/1, Vector Concatenate3/3
  DCM_B/N/1 -> calculating A_B/L/2(A_B/N)

== system SAD_project/Dynamics e Kinematics/DCM composition from quaternions 1 ==
  q(4x1) : Inport
  Cross product matrix composition : Subsystem
  Demux : Demux
  Dot Product : DotProduct  OutDataTypeStr=Inherit: Inherit via internal rule
  Gain : Gain  Gain=[1 0 0; 0 1 0; 0 0 1]
  Gain1 : Gain  Gain=2
  Gain2 : Gain  Gain=-2
  Mux : Mux  Inputs=3
  Product : Product  Multiplication=Matrix(*)
  Product1 : Product
  Square : Math  Operator=square
  Sum : Sum  Inputs=|-+
  Sum1 : Sum  Inputs=+++
  Transpose : Math  Operator=transpose
  DCM : Outport
  wires:
  Gain/1 -> Sum1/1
  Demux/1 -> Mux/1
  q(4x1)/1 -> Demux/1
  Demux/2 -> Mux/2
  Mux/1 -> Dot Product/2, Dot Product/1, Product/1, Cross product matrix composition/1(q_vect), Transpose/1  "q_vect"
  Demux/4 -> Gain2/1, Square/1  "q4"
  Demux/3 -> Mux/3
  Dot Product/1 -> Sum/1
  Sum/1 -> Gain/1
  Square/1 -> Sum/2
  Transpose/1 -> Product/2
  Product/1 -> Gain1/1
  Gain2/1 -> Product1/2
  Cross product matrix composition/1(q_vect cross) -> Product1/1  "omega_mat"
  Product1/1 -> Sum1/3
  Gain1/1 -> Sum1/2
  Sum1/1 -> DCM/1

== system SAD_project/Dynamics e Kinematics/Kinematics quaternion2 ==
  omega : Inport
  q0 : Inport  Port=2
  Demux : Demux
  Divide : Product  Inputs=*/
  Gain1 : Gain  Gain=-1
  Gain2 : Gain  Gain=-1
  Gain3 : Gain  Gain=1/2
  Gain4 : Gain  Gain=-1
  Integrator : Integrator  InitialConditionSource=external
  Matrix Multiply : Product  Multiplication=Matrix(*)
  Matrix OMEGA : Subsystem
  Mux : Mux
  Normalize Vector2 : Subsystem
  q : Outport
  q^(-1) : Outport  Port=2
  wires:
  Gain3/1 -> Matrix Multiply/1
  Matrix Multiply/1 -> Integrator/1
  omega/1 -> Matrix OMEGA/1(omega)
  Integrator/1 -> Normalize Vector2/1(Vector), Divide/1, Demux/1, q/1
  Matrix OMEGA/1(Matrix Omega) -> Gain3/1
  q0/1 -> Integrator/2
  Demux/2 -> Gain1/1
  Demux/3 -> Gain2/1
  Demux/4 -> Gain4/1
  Gain1/1 -> Mux/2
  Gain2/1 -> Mux/3
  Gain4/1 -> Mux/4
  Demux/1 -> Mux/1
  Mux/1 -> q^(-1)/1
  Normalize Vector2/1(Norm) -> Divide/2
  Divide/1 -> Matrix Multiply/2

== system SAD_project/Dynamics e Kinematics/Single spin dynamics ==
  Inertia matrix inverse : Inport
  Inertia matrix : Inport  Port=2
  Omega_0 : Inport  Port=3
  M : Inport  Port=4
  Cross Product : matrix_library/Cross Product
  Integrator1 : Integrator  InitialConditionSource=external
  Product : Product  Multiplication=Matrix(*)
  Product1 : Product  Multiplication=Matrix(*)
  Scope2 : Scope
  Sum : Sum  Inputs=|++
  Transpose1 : Math  Operator=transpose
  Omega : Outport
  wires:
  Transpose1/1 -> Omega/1
  Inertia matrix inverse/1 -> Product/1
  Integrator1/1 -> Product1/2, Transpose1/1, Cross Product/2, Scope2/1  "omega"
  Product/1 -> Integrator1/1  "omega_dot"
  Omega_0/1 -> Integrator1/2
  Product1/1 -> Cross Product/1
  Inertia matrix/1 -> Product1/1
  Cross Product/1 -> Sum/1
  Sum/1 -> Product/2
  M/1 -> Sum/2

== system SAD_project/Horizon Sensor/Normalize Vector1 ==
  Vector : Inport
  Divide : Product  Inputs=*/
  Normalize Vector : Subsystem  AncestorBlock=LibrarySAD5/Normalize Vector1
  Versor : Outport
  wires:
  Vector/1 -> Normalize Vector/1(Vector), Divide/1
  Divide/1 -> Versor/1
  Normalize Vector/1(Norm) -> Divide/2

== system SAD_project/Horizon Sensor/True Roll and Pitch betwen nadir and -z_body ==
  cone_limit_angle : Inport
  R_b : Inport  Port=2
  Abs : Abs  SaturateOnIntegerOverflow=off
  Abs1 : Abs  SaturateOnIntegerOverflow=off
  Asin : Trigonometry  Operator=asin
  Asin1 : Trigonometry  Operator=asin
  By defintion : Gain  Gain=-1
  Dot Product : DotProduct  OutDataTypeStr=Inherit: Inherit via internal rule
  Dot Product1 : DotProduct  OutDataTypeStr=Inherit: Inherit via internal rule
  Equal : RelationalOperator  Operator=>  OutDataTypeStr=boolean  RndMeth=Simplest  InputSameDT=off
  Equal1 : RelationalOperator  Operator=>  OutDataTypeStr=boolean  RndMeth=Simplest  InputSameDT=off
  NOT : Logic  Operator=NOT  IconShape=distinctive  AllPortsSameDT=off  OutDataTypeStr=boolean
  OR : Logic  Operator=OR  IconShape=distinctive  AllPortsSameDT=off  OutDataTypeStr=boolean
  Radians to Degrees : simulink_extras/Transformations/Radians to Degrees
  Radians to Degrees1 : simulink_extras/Transformations/Radians to Degrees
  x_b in body frame : Constant  Value=[1,0,0]'
  y_b in body frame1 : Constant  Value=[0,1,0]'
  Pitch : Outport
  Roll : Outport  Port=2
  Flag SensorSeeEarth : Outport  Port=3
  wires:
  Equal/1 -> OR/1
  Dot Product1/1 -> Asin1/1
  R_b/1 -> Dot Product1/2, Dot Product/2
  x_b in body frame/1 -> Dot Product/1
  y_b in body frame1/1 -> Dot Product1/1
  Dot Product/1 -> Asin/1
  By defintion/1 -> Radians to Degrees/1, Abs/1
  Asin/1 -> By defintion/1
  Asin1/1 -> Abs1/1, Radians to Degrees1/1
  Radians to Degrees1/1 -> Roll/1
  Abs1/1 -> Equal1/1
  Radians to Degrees/1 -> Pitch/1
  Abs/1 -> Equal/1
  cone_limit_angle/1 -> Equal/2, Equal1/2  "cone max angle"
  Equal1/1 -> OR/2
  OR/1 -> NOT/1
  NOT/1 -> Flag SensorSeeEarth/1

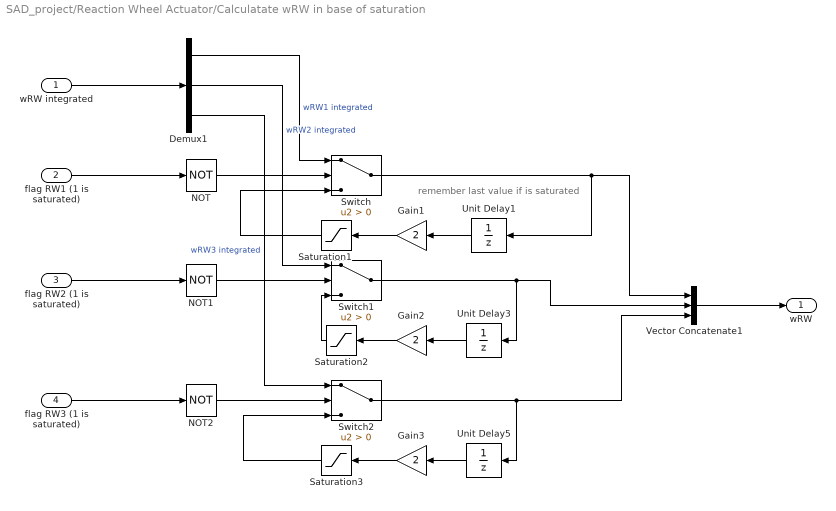
== system SAD_project/Reaction Wheel Actuator/Calculatate wRW in base of saturation ==
  note: remember last value if is saturated
  wRW integrated : Inport
  flag RW1 (1 is saturated) : Inport  Port=2
  flag RW2 (1 is saturated) : Inport  Port=3
  flag RW3 (1 is saturated) : Inport  Port=4
  Demux1 : Demux  Outputs=3
  Gain1 : Gain  Gain=2
  Gain2 : Gain  Gain=2
  Gain3 : Gain  Gain=2
  NOT : Logic  Operator=NOT  IconShape=distinctive  AllPortsSameDT=off  OutDataTypeStr=boolean
  NOT1 : Logic  Operator=NOT  IconShape=distinctive  AllPortsSameDT=off  OutDataTypeStr=boolean
  NOT2 : Logic  Operator=NOT  IconShape=distinctive  AllPortsSameDT=off  OutDataTypeStr=boolean
  Saturation1 : Saturate  UpperLimit=wMax_RW  LowerLimit=-wMax_RW
  Saturation2 : Saturate  UpperLimit=wMax_RW  LowerLimit=-wMax_RW
  Saturation3 : Saturate  UpperLimit=wMax_RW  LowerLimit=-wMax_RW
  Switch : Switch  Criteria=u2 > Threshold  SaturateOnIntegerOverflow=off  InputSameDT=off
  Switch1 : Switch  Criteria=u2 > Threshold  SaturateOnIntegerOverflow=off  InputSameDT=off
  Switch2 : Switch  Criteria=u2 > Threshold  SaturateOnIntegerOverflow=off  InputSameDT=off
  Unit Delay1 : UnitDelay  SampleTime=-1  HasFrameUpgradeWarning=on
  Unit Delay3 : UnitDelay  SampleTime=-1  HasFrameUpgradeWarning=on
  Unit Delay5 : UnitDelay  SampleTime=-1  HasFrameUpgradeWarning=on
  Vector Concatenate1 : Concatenate  NumInputs=3
  wRW : Outport
  wires:
  Gain2/1 -> Saturation2/1
  Switch1/1 -> Unit Delay3/1, Vector Concatenate1/2
  NOT/1 -> Switch/2
  flag RW1 (1 is saturated)/1 -> NOT/1
  Saturation3/1 -> Switch2/3
  NOT1/1 -> Switch1/2
  Saturation2/1 -> Switch1/3
  wRW integrated/1 -> Demux1/1
  Switch2/1 -> Unit Delay5/1, Vector Concatenate1/3
  Unit Delay5/1 -> Gain3/1
  Unit Delay3/1 -> Gain2/1
  Demux1/2 -> Switch1/1  "wRW2 integrated"
  Gain1/1 -> Saturation1/1
  Vector Concatenate1/1 -> wRW/1
  Switch/1 -> Unit Delay1/1, Vector Concatenate1/1
  Unit Delay1/1 -> Gain1/1
  Saturation1/1 -> Switch/3
  Demux1/3 -> Switch2/1  "wRW3 integrated"
  Demux1/1 -> Switch/1  "wRW1 integrated"
  NOT2/1 -> Switch2/2
  Gain3/1 -> Saturation3/1
  flag RW3 (1 is saturated)/1 -> NOT2/1
  flag RW2 (1 is saturated)/1 -> NOT1/1

== system SAD_project/Reaction Wheel Actuator/Subsystem1 ==
  h_r dot : Inport
  flag RW1 (1 is saturated) : Inport  Port=2
  flag RW2 (1 is saturated) : Inport  Port=3
  flag RW3 (1 is saturated) : Inport  Port=4
  Constant10 : Constant  Value=0
  Constant11 : Constant  Value=0
  Constant7 : Constant  Value=0
  Demux3 : Demux  Outputs=3
  Switch1 : Switch  Criteria=u2 > Threshold  SaturateOnIntegerOverflow=off  InputSameDT=off
  Switch2 : Switch  Criteria=u2 > Threshold  SaturateOnIntegerOverflow=off  InputSameDT=off
  Switch3 : Switch  Criteria=u2 > Threshold  SaturateOnIntegerOverflow=off  InputSameDT=off
  Vector Concatenate2 : Concatenate  NumInputs=3
  M : Outport
  wires:
  Demux3/3 -> Switch2/3
  Constant11/1 -> Switch2/1
  Switch2/1 -> Vector Concatenate2/3
  Demux3/1 -> Switch3/3
  Demux3/2 -> Switch1/3
  Switch3/1 -> Vector Concatenate2/1
  Switch1/1 -> Vector Concatenate2/2
  flag RW3 (1 is saturated)/1 -> Switch2/2
  Constant7/1 -> Switch3/1
  Constant10/1 -> Switch1/1
  flag RW1 (1 is saturated)/1 -> Switch3/2
  h_r dot/1 -> Demux3/1
  flag RW2 (1 is saturated)/1 -> Switch1/2
  Vector Concatenate2/1 -> M/1

== system SAD_project/Reaction Wheel Actuator/detect if the RW is saturated (output == 1 isSaturated) ==
  w : Inport
  Abs : Abs  SaturateOnIntegerOverflow=off
  Compare To Constant : simulink/Logic and Bit Operations/Compare To Constant  relop=>=  const=wMax_RW  OutDataTypeStr=boolean
  Demux : Demux  Outputs=3
  Logical Operator : Logic  Operator=OR  AllPortsSameDT=off  OutDataTypeStr=boolean
  Logical Operator1 : Logic  Operator=OR  AllPortsSameDT=off  OutDataTypeStr=boolean
  Logical Operator2 : Logic  Operator=OR  AllPortsSameDT=off  OutDataTypeStr=boolean
  Unit Delay : UnitDelay  SampleTime=-1  HasFrameUpgradeWarning=on
  Unit Delay2 : UnitDelay  SampleTime=-1  HasFrameUpgradeWarning=on
  Unit Delay4 : UnitDelay  SampleTime=-1  HasFrameUpgradeWarning=on
  flag RW1 : Outport
  flag RW2 : Outport  Port=2
  flag RW3 : Outport  Port=3
  wires:
  Unit Delay4/1 -> Logical Operator2/2
  Unit Delay/1 -> Logical Operator/2
  Demux/1 -> Logical Operator/1
  Logical Operator/1 -> flag RW1/1, Unit Delay/1
  Unit Delay2/1 -> Logical Operator1/2
  Logical Operator2/1 -> flag RW3/1, Unit Delay4/1
  Demux/2 -> Logical Operator1/1
  Logical Operator1/1 -> flag RW2/1, Unit Delay2/1
  Demux/3 -> Logical Operator2/1
  Abs/1 -> Compare To Constant/1
  w/1 -> Abs/1
  Compare To Constant/1 -> Demux/1

== system SAD_project/Statistical methods attitude determination (quaternion  Wabha’s problem) /For Iterator Subsystem to calculate B matrix ==
  note: Remember the last matrix B
  note: count the index
      | Important to flag reset in "State variable" to reset unit delay
  note: It's a for loop that resolve this expression
      | 𝐵 = ∑ 𝛼_𝑖*𝑠_𝑖*𝑣_𝑖' = [𝑏ij] to obatain matix B that it is a square matrix of order 3
      |
      | Analogous code for the iteration:
      |
      | for i = 1:size(alpha,2)
      | B = B + alpha(i)*s(:,i)*v(:,i)'
      | end
  alpha : Inport
  s matrix : Inport  Port=2
  v matrix : Inport  Port=3
  Add : Sum
  For Iterator : ForIterator  ResetStates=reset  IterationLimit=size(alpha,2)
  Matrix Multiply : Product  Multiplication=Matrix(*)
  Product : Product
  Transpose : Math  Operator=transpose
  Unit Delay1 : UnitDelay  SampleTime=-1  HasFrameUpgradeWarning=on
  Variable Selector : dspindex/Variable Selector  NumInputs=1  rowsOrCols=Columns  IdxMode=Variable  Elements=[1 3]  ZerOneIdxMode=One-based  errmode=Clip Index  FillMode=on  FillValues=0
  Variable Selector1 : dspindex/Variable Selector  NumInputs=1  rowsOrCols=Columns  IdxMode=Variable  Elements=[1 3]  ZerOneIdxMode=One-based  errmode=Clip Index  FillMode=on  FillValues=0
  Variable Selector2 : dspindex/Variable Selector  NumInputs=1  rowsOrCols=Columns  IdxMode=Variable  Elements=[1 3]  ZerOneIdxMode=One-based  errmode=Clip Index  FillMode=on  FillValues=0
  B matrix : Outport
  wires:
  For Iterator/1 -> Variable Selector1/2, Variable Selector/2, Variable Selector2/2
  alpha/1 -> Variable Selector2/1
  s matrix/1 -> Variable Selector/1
  Variable Selector2/1 -> Product/1
  Variable Selector/1 -> Product/2
  Product/1 -> Matrix Multiply/1
  Variable Selector1/1 -> Transpose/1
  Transpose/1 -> Matrix Multiply/2
  Matrix Multiply/1 -> Add/1
  v matrix/1 -> Variable Selector1/1
  Unit Delay1/1 -> Add/2
  Add/1 -> Unit Delay1/1, B matrix/1

== system SAD_project/Statistical methods attitude determination (quaternion  Wabha’s problem) /Matrix trace ==
  Matrix : Inport
  Extract Diagonal : matrix_library/Extract Diagonal
      settings: LibrarySourceBlock=|
      | simulink/Matrix
      | Operations/Extract Diagonal
  Sum of Elements : Sum  Inputs=+
  trace : Outport
  wires:
  Extract Diagonal/1 -> Sum of Elements/1
  Sum of Elements/1 -> trace/1  "sigma"
  Matrix/1 -> Extract Diagonal/1
